simulink model "Filialist_PORTSDONE"  (R2019b)
settings: Solver=FixedStepAuto  StartTime=0.0  StopTime=inf  RelTol=1e-3
libraries: vexarmcortexlib x26, vexcommonlib x7
settings Model: ExtModeTrigDuration=25  Creator=nicoa  LastModifiedBy=nicoa
settings OptimizationCC: EnhancedBackFolding=on  PassReuseOutputArgsAs=Individual arguments  ZeroExternalMemoryAtStartup=off  ZeroInternalMemoryAtStartup=off  MaxStackSize=64  OptimizeBlockOrder=speed  DifferentSizesBufferReuse=on  OptimizationCustomize=off  EfficientTunableParamExpr=on
settings DebuggingCC: ParameterTunabilityLossMsg=error
settings HardwareCC: ProdBitPerPointer=32  ProdBitPerSizeT=32  ProdBitPerPtrDiffT=32  ProdLargestAtomicInteger=Long  ProdLargestAtomicFloat=Double  ProdWordSize=32  ProdHWDeviceType=ARM Compatible->ARM Cortex
settings SFSimCC: MATLABDynamicMemAlloc=off
settings RTWCC: SystemTargetFile=ert.tlc  HardwareBoard=ARM Cortex-based VEX Microcontroller  TLCOptions="-aInlineSetEventsForThisBaseRateFcn=TLC_FALSE -aSuppressMultiTaskScheduler=TLC_FALSE  -aRateBasedStepFcn=0"  TemplateMakefile=ert_default_tmf  GenerateReport=on  Toolchain=GNU Tools for VEX ARM Cortex  IncludeHyperlinkInReport=on  LaunchReport=on  GenerateTraceInfo=on  GenerateTraceReport=on  GenerateTraceReportSl=on  GenerateTraceReportSf=on  GenerateTraceReportEml=on
settings CodeAppCC: ForceParamTrailComments=on  IgnoreCustomStorageClasses=off  OperatorAnnotations=on  SimulinkDataObjDesc=on  SFDataObjDesc=on  InsertBlockDesc=on

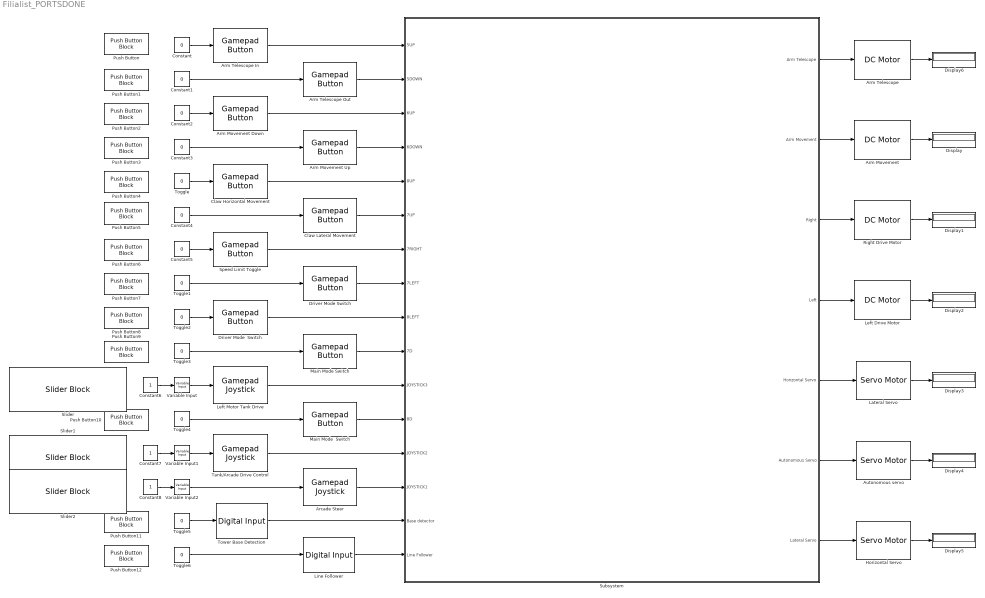
== system Filialist_PORTSDONE ==
  "Arcade Steer " : vexarmcortexlib/Gamepad/Gamepad Joystick  joystick=1  chan=1  SimulationIn=on  SampleTime=0.02
      settings: SourceProductName=Simulink Coder Support Package for ARM Cortex-based VEX Microcontroller  SourceProductBaseCode=EC_VEX_MICRO
  Arm Movement : vexarmcortexlib/Actuators/DC Motor  motor=6  scaleFactor=1/13.5  SimulationOut=on
      settings: SourceProductName=Simulink Coder Support Package for ARM Cortex-based VEX Microcontroller  SourceProductBaseCode=EC_VEX_MICRO
  Arm Movement Down : vexarmcortexlib/Gamepad/Gamepad Button  joystick=1  chan=6  button56=Down  button78=Down  SimulationIn=on  SampleTime=0.02
      settings: SourceProductName=Simulink Coder Support Package for ARM Cortex-based VEX Microcontroller  SourceProductBaseCode=EC_VEX_MICRO
  Arm Movement Up : vexarmcortexlib/Gamepad/Gamepad Button  joystick=1  chan=6  button56=Up  button78=Down  SimulationIn=on  SampleTime=0.02
      settings: SourceProductName=Simulink Coder Support Package for ARM Cortex-based VEX Microcontroller  SourceProductBaseCode=EC_VEX_MICRO
  Arm Telescope : vexarmcortexlib/Actuators/DC Motor  motor=2  scaleFactor=1/13.5  SimulationOut=on
      settings: SourceProductName=Simulink Coder Support Package for ARM Cortex-based VEX Microcontroller  SourceProductBaseCode=EC_VEX_MICRO
  Arm Telescope In : vexarmcortexlib/Gamepad/Gamepad Button  joystick=1  chan=5  button56=Down  button78=Down  SimulationIn=on  SampleTime=0.02
      settings: SourceProductName=Simulink Coder Support Package for ARM Cortex-based VEX Microcontroller  SourceProductBaseCode=EC_VEX_MICRO
  Arm Telescope Out : vexarmcortexlib/Gamepad/Gamepad Button  joystick=1  chan=5  button56=Up  button78=Down  SimulationIn=on  SampleTime=0.02
      settings: SourceProductName=Simulink Coder Support Package for ARM Cortex-based VEX Microcontroller  SourceProductBaseCode=EC_VEX_MICRO
  Autonomous servo : vexarmcortexlib/Actuators/Servo Motor  motor=5  scaleFactor=60/127  SimulationOut=on
      settings: SourceProductName=Simulink Coder Support Package for ARM Cortex-based VEX Microcontroller  SourceProductBaseCode=EC_VEX_MICRO
  Claw Horizontal Movement : vexarmcortexlib/Gamepad/Gamepad Button  joystick=1  chan=8  button56=Up  button78=Up  SimulationIn=on  SampleTime=0.02
      settings: SourceProductName=Simulink Coder Support Package for ARM Cortex-based VEX Microcontroller  SourceProductBaseCode=EC_VEX_MICRO
  Claw Lateral Movement : vexarmcortexlib/Gamepad/Gamepad Button  joystick=1  chan=7  button56=Up  button78=Up  SimulationIn=on  SampleTime=0.02
      settings: SourceProductName=Simulink Coder Support Package for ARM Cortex-based VEX Microcontroller  SourceProductBaseCode=EC_VEX_MICRO
  Constant{,1..5} (6 alike) : Constant  Value=0
  Constant6 : Constant
  Constant7 : Constant
  Constant8 : Constant
  Display{,1..6} (7 alike) : Display
  Driver Mode  Switch : vexarmcortexlib/Gamepad/Gamepad Button  joystick=1  chan=8  button56=Up  button78=Left  SimulationIn=on  SampleTime=0.02
      settings: SourceProductName=Simulink Coder Support Package for ARM Cortex-based VEX Microcontroller  SourceProductBaseCode=EC_VEX_MICRO
  Driver Mode Switch : vexarmcortexlib/Gamepad/Gamepad Button  joystick=1  chan=7  button56=Up  button78=Left  SimulationIn=on  SampleTime=0.02
      settings: SourceProductName=Simulink Coder Support Package for ARM Cortex-based VEX Microcontroller  SourceProductBaseCode=EC_VEX_MICRO
  Horizontal Servo : vexarmcortexlib/Actuators/Servo Motor  motor=3  scaleFactor=60/127  SimulationOut=on
      settings: SourceProductName=Simulink Coder Support Package for ARM Cortex-based VEX Microcontroller  SourceProductBaseCode=EC_VEX_MICRO
  Lateral Servo : vexarmcortexlib/Actuators/Servo Motor  motor=8  scaleFactor=60/127  SimulationOut=on
      settings: SourceProductName=Simulink Coder Support Package for ARM Cortex-based VEX Microcontroller  SourceProductBaseCode=EC_VEX_MICRO
  "Left Drive Motor " : vexarmcortexlib/Actuators/DC Motor  motor=9  scaleFactor=1/13.5  SimulationOut=on
      settings: SourceProductName=Simulink Coder Support Package for ARM Cortex-based VEX Microcontroller  SourceProductBaseCode=EC_VEX_MICRO
  Left Motor Tank Drive : vexarmcortexlib/Gamepad/Gamepad Joystick  joystick=1  chan=3  SimulationIn=on  SampleTime=0.02
      settings: SourceProductName=Simulink Coder Support Package for ARM Cortex-based VEX Microcontroller  SourceProductBaseCode=EC_VEX_MICRO
  Line Follower : vexarmcortexlib/Sensors/Digital Input  inChan=1  SimulationIn=on  SampleTime=0.2
      settings: SourceProductName=Simulink Coder Support Package for ARM Cortex-based VEX Microcontroller  SourceProductBaseCode=EC_VEX_MICRO
  Main Mode  Switch : vexarmcortexlib/Gamepad/Gamepad Button  joystick=1  chan=8  button56=Up  button78=Down  SimulationIn=on  SampleTime=0.02
      settings: SourceProductName=Simulink Coder Support Package for ARM Cortex-based VEX Microcontroller  SourceProductBaseCode=EC_VEX_MICRO
  Main Mode Switch : vexarmcortexlib/Gamepad/Gamepad Button  joystick=1  chan=7  button56=Up  button78=Down  SimulationIn=on  SampleTime=0.02
      settings: SourceProductName=Simulink Coder Support Package for ARM Cortex-based VEX Microcontroller  SourceProductBaseCode=EC_VEX_MICRO
  Push Button{,1..12} (13 alike) : PushButtonBlock
  Right Drive Motor : vexarmcortexlib/Actuators/DC Motor  motor=4  scaleFactor=1/13.5  SimulationOut=on
      settings: SourceProductName=Simulink Coder Support Package for ARM Cortex-based VEX Microcontroller  SourceProductBaseCode=EC_VEX_MICRO
  Slider : SliderBlock  LabelPosition=Hide  ScaleMin=-127  ScaleMax=127
  Slider1 : SliderBlock  LabelPosition=Hide  ScaleMin=-127  ScaleMax=127
  Slider2 : SliderBlock  LabelPosition=Hide  ScaleMin=-127  ScaleMax=127
  Speed Limit Toggle : vexarmcortexlib/Gamepad/Gamepad Button  joystick=1  chan=7  button56=Up  button78=Right  SimulationIn=on  SampleTime=0.02
      settings: SourceProductName=Simulink Coder Support Package for ARM Cortex-based VEX Microcontroller  SourceProductBaseCode=EC_VEX_MICRO
  Subsystem : Subsystem
  Tank/Arcade Drive Control : vexarmcortexlib/Gamepad/Gamepad Joystick  joystick=1  chan=2  SimulationIn=on  SampleTime=0.02
      settings: SourceProductName=Simulink Coder Support Package for ARM Cortex-based VEX Microcontroller  SourceProductBaseCode=EC_VEX_MICRO
  Toggle{,1..6} (7 alike) : Constant  Value=0
      settings: OpenFcn=|
      | if strcmp('0',get_param(gcb, 'Value'))                        set_param(gcb, 'Value', '1');
      | else
      |             set_param(gcb, 'Value', '0');
      | end
  Tower Base Detection : vexarmcortexlib/Sensors/Digital Input  inChan=11  SimulationIn=on  SampleTime=0.2
      settings: SourceProductName=Simulink Coder Support Package for ARM Cortex-based VEX Microcontroller  SourceProductBaseCode=EC_VEX_MICRO
  Variable Input : vexarmcortexlib/Utilities/Variable Input  low=-127  gain=0  high=127
      settings: SourceProductName=Simulink Coder Support Package for ARM Cortex-based VEX Microcontroller  SourceProductBaseCode=EC_VEX_MICRO
  Variable Input1 : vexarmcortexlib/Utilities/Variable Input  low=-127  gain=0  high=127
      settings: SourceProductName=Simulink Coder Support Package for ARM Cortex-based VEX Microcontroller  SourceProductBaseCode=EC_VEX_MICRO
  Variable Input2 : vexarmcortexlib/Utilities/Variable Input  low=-127  gain=0  high=127
      settings: SourceProductName=Simulink Coder Support Package for ARM Cortex-based VEX Microcontroller  SourceProductBaseCode=EC_VEX_MICRO
  wires:
  Main Mode  Switch/1 -> Subsystem/12(8D)
  Main Mode Switch/1 -> Subsystem/10(7D)
  Subsystem/4(Left) -> "Left Drive Motor "/1
  Subsystem/6(Autonomous Servo) -> Autonomous servo/1
  Tower Base Detection/1 -> Subsystem/15(Base detector)
  Line Follower/1 -> Subsystem/16(Line Follower)
  Driver Mode  Switch/1 -> Subsystem/9(8LEFT)
  Driver Mode Switch/1 -> Subsystem/8(7LEFT)
  Speed Limit Toggle/1 -> Subsystem/7(7RIGHT)
  Tank/Arcade Drive Control/1 -> Subsystem/13(JOYSTICK2)
  Left Motor Tank Drive/1 -> Subsystem/11(JOYSTICK3)
  "Arcade Steer "/1 -> Subsystem/14(JOYSTICK1)
  Subsystem/3(Right) -> Right Drive Motor/1
  Subsystem/7(Lateral Servo) -> Horizontal Servo/1
  Subsystem/5(Horizontal Servo) -> Lateral Servo/1
  Claw Lateral Movement/1 -> Subsystem/6(7UP)
  Claw Horizontal Movement/1 -> Subsystem/5(8UP)
  Subsystem/2(Arm Movement) -> Arm Movement/1
  Arm Movement Up/1 -> Subsystem/4(6DOWN)
  Arm Movement Down/1 -> Subsystem/3(6UP)
  Subsystem/1(Arm Telescope) -> Arm Telescope/1
  Arm Telescope Out/1 -> Subsystem/2(5DOWN)
  Arm Telescope In/1 -> Subsystem/1(5UP)
  Arm Movement/1 -> Display/1
  Right Drive Motor/1 -> Display1/1
  "Left Drive Motor "/1 -> Display2/1
  Lateral Servo/1 -> Display3/1
  Autonomous servo/1 -> Display4/1
  Horizontal Servo/1 -> Display5/1
  Arm Telescope/1 -> Display6/1
  Constant/1 -> Arm Telescope In/1
  Constant1/1 -> Arm Telescope Out/1
  Constant2/1 -> Arm Movement Down/1
  Constant3/1 -> Arm Movement Up/1
  Toggle/1 -> Claw Horizontal Movement/1
  Constant4/1 -> Claw Lateral Movement/1
  Constant5/1 -> Speed Limit Toggle/1
  Toggle1/1 -> Driver Mode Switch/1
  Toggle2/1 -> Driver Mode  Switch/1
  Toggle3/1 -> Main Mode Switch/1
  Constant6/1 -> Variable Input/1
  Variable Input/1 -> Left Motor Tank Drive/1
  Variable Input1/1 -> Tank/Arcade Drive Control/1
  Constant7/1 -> Variable Input1/1
  Variable Input2/1 -> "Arcade Steer "/1
  Constant8/1 -> Variable Input2/1
  Toggle4/1 -> Main Mode  Switch/1
  Toggle5/1 -> Tower Base Detection/1
  Toggle6/1 -> Line Follower/1

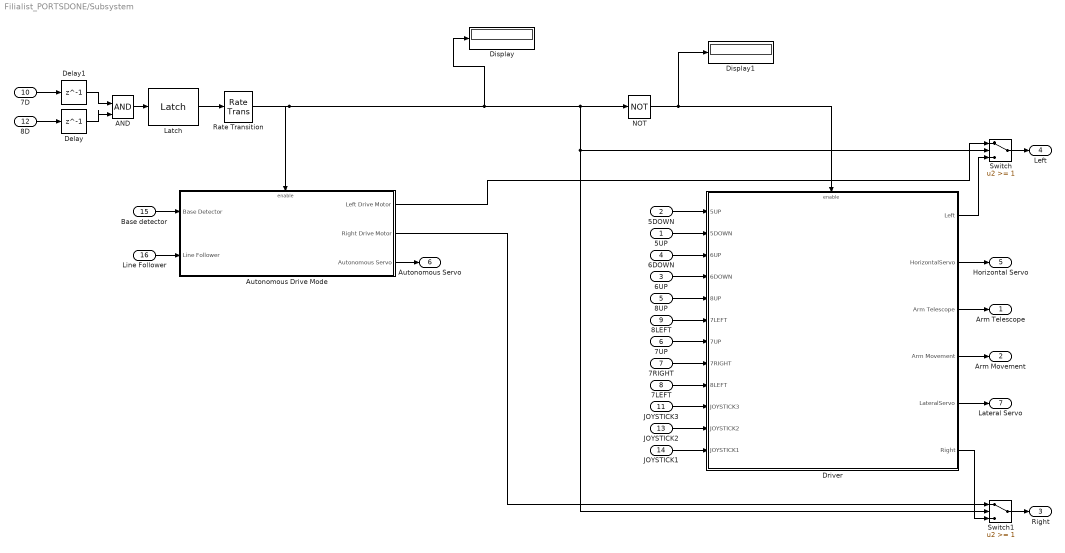
== system Filialist_PORTSDONE/Subsystem ==
  5UP : Inport
  5DOWN : Inport  Port=2
  6UP : Inport  Port=3
  6DOWN : Inport  Port=4
  8UP : Inport  Port=5
  7UP : Inport  Port=6
  7RIGHT : Inport  Port=7
  7LEFT : Inport  Port=8
  8LEFT : Inport  Port=9
  7D : Inport  Port=10
  JOYSTICK3 : Inport  Port=11
  8D : Inport  Port=12
  JOYSTICK2 : Inport  Port=13
  JOYSTICK1 : Inport  Port=14
  Base detector : Inport  Port=15
  Line Follower : Inport  Port=16
  "AND " : Logic  IconShape=distinctive  AllPortsSameDT=off  OutDataTypeStr=boolean
  Autonomous Drive Mode : Subsystem
  Delay : Delay  DelayLength=1  InitialCondition=0  SampleTime=1
  Delay1 : Delay  DelayLength=1  InitialCondition=0  SampleTime=1
  Display : Display
  Display1 : Display
  Driver : Subsystem  TreatAsAtomicUnit=on
  Latch : vexcommonlib/Latch  output0=off  BlockPlatform=vexarmcortex
      settings: SourceProductName=Simulink Coder Support Package for ARM Cortex-based VEX Microcontroller  SourceProductBaseCode=EC_VEX_MICRO
  NOT : Logic  Operator=NOT  IconShape=distinctive  AllPortsSameDT=off  OutDataTypeStr=boolean
  Rate Transition : RateTransition
  Switch : Switch  Threshold=1
  Switch1 : Switch  Threshold=1
  Arm Telescope : Outport
  Arm Movement : Outport  Port=2
  Right : Outport  Port=3
  Left : Outport  Port=4
  Horizontal Servo : Outport  Port=5
  Autonomous Servo : Outport  Port=6
  Lateral Servo : Outport  Port=7
  wires:
  "AND "/1 -> Latch/1
  Delay1/1 -> "AND "/1
  Latch/1 -> Rate Transition/1
  7D/1 -> Delay1/1
  Delay/1 -> "AND "/2
  8D/1 -> Delay/1
  Autonomous Drive Mode/3(Autonomous Servo) -> Autonomous Servo/1
  Rate Transition/1 -> Autonomous Drive Mode/Enable, NOT/1, Switch1/2, Switch/2, Display/1
  NOT/1 -> Driver/Enable, Display1/1
  Autonomous Drive Mode/1(Left Drive Motor) -> Switch/1
  Switch/1 -> Left/1
  Autonomous Drive Mode/2(Right Drive Motor) -> Switch1/1
  Switch1/1 -> Right/1
  Line Follower/1 -> Autonomous Drive Mode/2(Line Follower)
  Base detector/1 -> Autonomous Drive Mode/1(Base Detector)
  7LEFT/1 -> Driver/9(8LEFT)
  8LEFT/1 -> Driver/6(7LEFT)
  7RIGHT/1 -> Driver/8(7RIGHT)
  JOYSTICK3/1 -> Driver/10(JOYSTICK3)
  JOYSTICK2/1 -> Driver/11(JOYSTICK2)
  JOYSTICK1/1 -> Driver/12(JOYSTICK1)
  Driver/5(LateralServo) -> Lateral Servo/1
  Driver/2(HorizontalServo) -> Horizontal Servo/1
  8UP/1 -> Driver/5(8UP)
  7UP/1 -> Driver/7(7UP)
  Driver/4(Arm Movement) -> Arm Movement/1
  6UP/1 -> Driver/4(6DOWN)
  6DOWN/1 -> Driver/3(6UP)
  Driver/3(Arm Telescope) -> Arm Telescope/1
  5UP/1 -> Driver/2(5DOWN)
  5DOWN/1 -> Driver/1(5UP)
  Driver/6(Right) -> Switch1/3
  Driver/1(Left) -> Switch/3

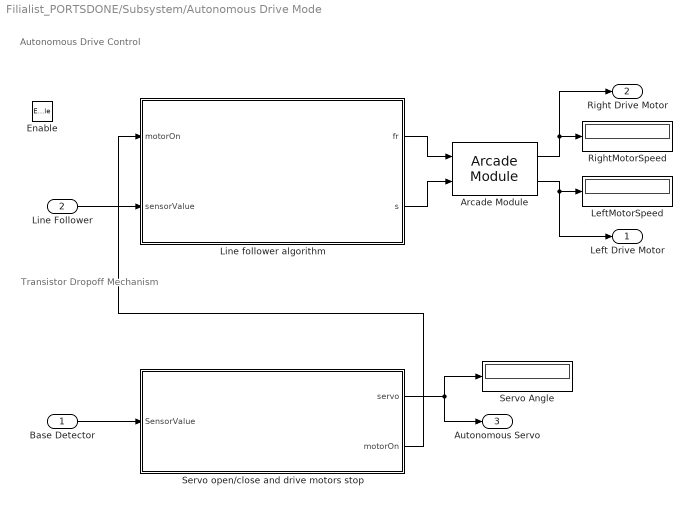
== system Filialist_PORTSDONE/Subsystem/Autonomous Drive Mode ==
  note: Transistor Dropoff Mechanism
  note: Autonomous Drive Control
  Base Detector : Inport
  Line Follower : Inport  Port=2
  Enable : EnablePort
  Arcade Module : vexcommonlib/Arcade Module  BlockPlatform=vexarmcortex
      settings: SourceProductName=Simulink Coder Support Package for ARM Cortex-based VEX Microcontroller  SourceProductBaseCode=EC_VEX_MICRO
  LeftMotorSpeed : Display
  Line follower algorithm : Stateflow chart  TreatAsAtomicUnit=on
  RightMotorSpeed : Display
  Servo Angle : Display
  Servo open/close and drive motors stop : Stateflow chart  TreatAsAtomicUnit=on
  Left Drive Motor : Outport
  Right Drive Motor : Outport  Port=2
  Autonomous Servo : Outport  Port=3
  wires:
  Base Detector/1 -> Servo open/close and drive motors stop/1(SensorValue)
  Line Follower/1 -> Line follower algorithm/2(sensorValue)
  Line follower algorithm/2(s) -> Arcade Module/2
  Line follower algorithm/1(fr) -> Arcade Module/1
  Arcade Module/1 -> RightMotorSpeed/1, Right Drive Motor/1
  Arcade Module/2 -> LeftMotorSpeed/1, Left Drive Motor/1
  Servo open/close and drive motors stop/1(servo) -> Autonomous Servo/1, Servo Angle/1
  Servo open/close and drive motors stop/2(motorOn) -> Line follower algorithm/1(motorOn)

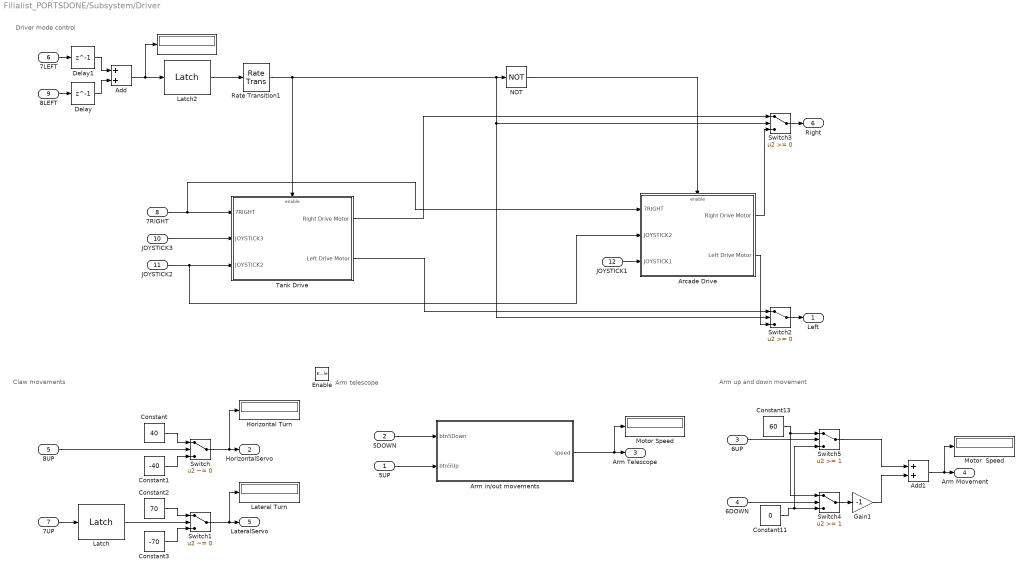
== system Filialist_PORTSDONE/Subsystem/Driver ==
  note: Arm telescope
  note: Claw movements
  note: Arm up and down movement
  note: Driver mode control
  5UP : Inport
  5DOWN : Inport  Port=2
  6UP : Inport  Port=3
  6DOWN : Inport  Port=4
  8UP : Inport  Port=5
  7LEFT : Inport  Port=6
  7UP : Inport  Port=7
  7RIGHT : Inport  Port=8
  8LEFT : Inport  Port=9
  JOYSTICK3 : Inport  Port=10
  JOYSTICK2 : Inport  Port=11
  JOYSTICK1 : Inport  Port=12
  Enable : EnablePort
  " " : Display
  Add : Sum
  Add1 : Sum
  "Arcade Drive " : Subsystem  TreatAsAtomicUnit=on
  Arm in/out movements : Stateflow chart  BlockKeywords=__PRM__SERIALIZED__DATA__:Stateflow Chart,Stateflow Diagram  TreatAsAtomicUnit=on
  Constant : Constant  Value=40
  Constant1 : Constant  Value=-40
  Constant11 : Constant  Value=0
  Constant13 : Constant  Value=60
  Constant2 : Constant  Value=70
  Constant3 : Constant  Value=-70
  Delay : Delay  DelayLength=1  InitialCondition=0  SampleTime=1
  Delay1 : Delay  DelayLength=1  InitialCondition=0  SampleTime=1
  Gain1 : Gain  Gain=-1
  Horizontal Turn : Display
  Latch : vexcommonlib/Latch  output0=off  BlockPlatform=vexarmcortex
      settings: SourceProductName=Simulink Coder Support Package for ARM Cortex-based VEX Microcontroller  SourceProductBaseCode=EC_VEX_MICRO
  Latch2 : vexcommonlib/Latch  output0=off  BlockPlatform=vexarmcortex
      settings: SourceProductName=Simulink Coder Support Package for ARM Cortex-based VEX Microcontroller  SourceProductBaseCode=EC_VEX_MICRO
  Lateral Turn : Display
  Motor  Speed : Display
  Motor Speed : Display
  NOT : Logic  Operator=NOT  IconShape=distinctive  AllPortsSameDT=off  OutDataTypeStr=boolean
  Rate Transition1 : RateTransition
  Switch : Switch  Criteria=u2 ~= 0
  Switch1 : Switch  Criteria=u2 ~= 0
  Switch2 : Switch
  Switch3 : Switch
  Switch4 : Switch  Threshold=1
  Switch5 : Switch  Threshold=1
  "Tank Drive " : Subsystem  TreatAsAtomicUnit=on
  Left : Outport
  HorizontalServo : Outport  Port=2
  Arm Telescope : Outport  Port=3
  Arm Movement : Outport  Port=4
  LateralServo : Outport  Port=5
  Right : Outport  Port=6
  wires:
  Rate Transition1/1 -> Switch2/2, Switch3/2, NOT/1, "Tank Drive "/Enable
  7LEFT/1 -> Delay1/1
  NOT/1 -> "Arcade Drive "/Enable
  Delay1/1 -> Add/1
  Delay/1 -> Add/2
  Latch2/1 -> Rate Transition1/1
  Add/1 -> " "/1, Latch2/1
  8LEFT/1 -> Delay/1
  JOYSTICK3/1 -> "Tank Drive "/2(JOYSTICK3)
  JOYSTICK2/1 -> "Tank Drive "/3(JOYSTICK2), "Arcade Drive "/2(JOYSTICK2)
  JOYSTICK1/1 -> "Arcade Drive "/3(JOYSTICK1)
  Constant/1 -> Switch/1
  7UP/1 -> Latch/1
  Latch/1 -> Switch1/2
  Switch/1 -> Horizontal Turn/1, HorizontalServo/1
  Constant1/1 -> Switch/3
  Switch1/1 -> Lateral Turn/1, LateralServo/1
  Constant2/1 -> Switch1/1
  Constant3/1 -> Switch1/3
  Switch4/1 -> Gain1/1
  Constant11/1 -> Switch5/3, Switch4/3
  6DOWN/1 -> Switch4/2
  6UP/1 -> Switch5/2
  Constant13/1 -> Switch5/1, Switch4/1
  Add1/1 -> Motor  Speed/1, Arm Movement/1
  5UP/1 -> Arm in/out movements/2(btn5Up)
  Arm in/out movements/1(speed) -> Motor Speed/1, Arm Telescope/1
  5DOWN/1 -> Arm in/out movements/1(btn5Down)
  Switch2/1 -> Left/1
  "Arcade Drive "/2(Left Drive Motor) -> Switch2/3
  Switch3/1 -> Right/1
  "Arcade Drive "/1(Right Drive Motor) -> Switch3/3
  7RIGHT/1 -> "Tank Drive "/1(7RIGHT), "Arcade Drive "/1(7RIGHT)
  "Tank Drive "/2(Left Drive Motor) -> Switch2/1
  "Tank Drive "/1(Right Drive Motor) -> Switch3/1
  Switch5/1 -> Add1/1
  Gain1/1 -> Add1/2
  8UP/1 -> Switch/2

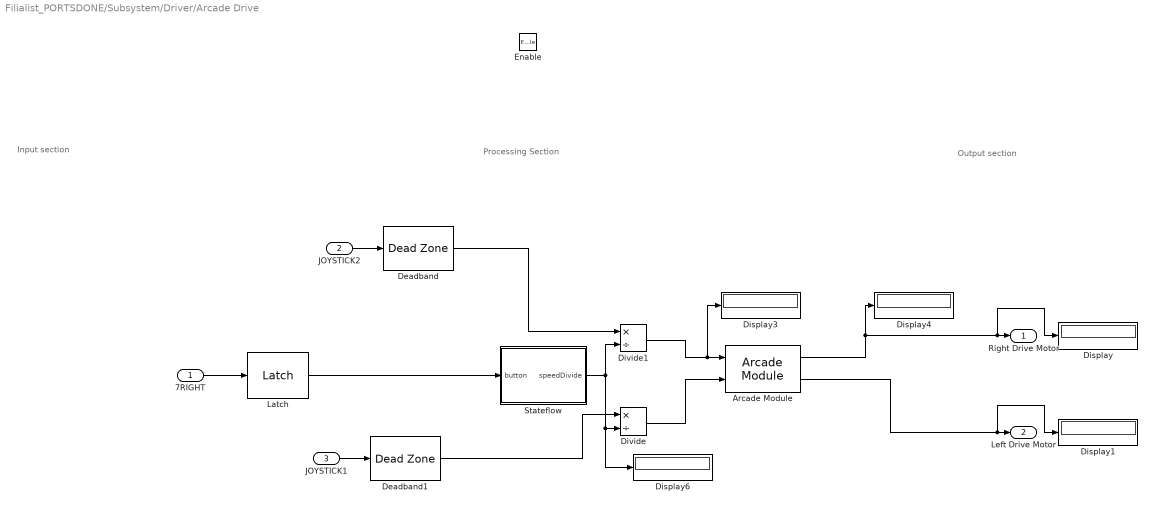
== system Filialist_PORTSDONE/Subsystem/Driver/Arcade Drive  ==
  note: Output section
  note: Processing Section
  note: Input section
  7RIGHT : Inport
  JOYSTICK2 : Inport  Port=2
  JOYSTICK1 : Inport  Port=3
  Enable : EnablePort
  Arcade Module : vexcommonlib/Arcade Module  BlockPlatform=vexarmcortex
      settings: SourceProductName=Simulink Coder Support Package for ARM Cortex-based VEX Microcontroller  SourceProductBaseCode=EC_VEX_MICRO
  Deadband : DeadZone  LowerValue=-5  UpperValue=5  SaturateOnIntegerOverflow=on
  Deadband1 : DeadZone  LowerValue=-5  UpperValue=5  SaturateOnIntegerOverflow=on
  Display{,1,3..4,6} (5 alike) : Display
  Divide : Product  Inputs=*/
  Divide1 : Product  Inputs=*/
  Latch : vexcommonlib/Latch  output0=off  BlockPlatform=vexarmcortex
      settings: SourceProductName=Simulink Coder Support Package for ARM Cortex-based VEX Microcontroller  SourceProductBaseCode=EC_VEX_MICRO
  Stateflow : Stateflow chart  TreatAsAtomicUnit=on
  Right Drive Motor : Outport
  Left Drive Motor : Outport  Port=2
  wires:
  JOYSTICK1/1 -> Deadband1/1
  JOYSTICK2/1 -> Deadband/1
  7RIGHT/1 -> Latch/1
  Stateflow/1(speedDivide) -> Display6/1, Divide/2, Divide1/2
  Deadband/1 -> Divide1/1
  Deadband1/1 -> Divide/1
  Divide/1 -> Arcade Module/2
  Divide1/1 -> Display3/1, Arcade Module/1
  Arcade Module/1 -> Display/1, Right Drive Motor/1, Display4/1
  Arcade Module/2 -> Display1/1, Left Drive Motor/1
  Latch/1 -> Stateflow/1(button)

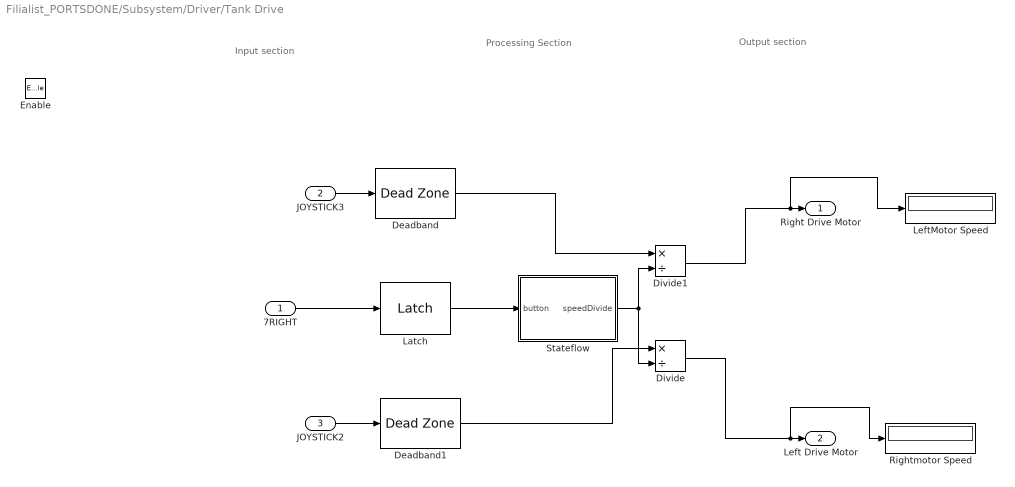
== system Filialist_PORTSDONE/Subsystem/Driver/Tank Drive  ==
  note: Output section
  note: Processing Section
  note: Input section
  7RIGHT : Inport
  JOYSTICK3 : Inport  Port=2
  JOYSTICK2 : Inport  Port=3
  Enable : EnablePort
  Deadband : DeadZone  LowerValue=-5  UpperValue=5  SaturateOnIntegerOverflow=on
  Deadband1 : DeadZone  LowerValue=-5  UpperValue=5  SaturateOnIntegerOverflow=on
  Divide : Product  Inputs=*/
  Divide1 : Product  Inputs=*/
  Latch : vexcommonlib/Latch  output0=off  BlockPlatform=vexarmcortex
      settings: SourceProductName=Simulink Coder Support Package for ARM Cortex-based VEX Microcontroller  SourceProductBaseCode=EC_VEX_MICRO
  LeftMotor Speed : Display
  Rightmotor Speed : Display
  Stateflow : Stateflow chart  TreatAsAtomicUnit=on
  Right Drive Motor : Outport
  Left Drive Motor : Outport  Port=2
  wires:
  JOYSTICK3/1 -> Deadband/1
  7RIGHT/1 -> Latch/1
  Latch/1 -> Stateflow/1(button)
  Stateflow/1(speedDivide) -> Divide1/2, Divide/2
  Deadband/1 -> Divide1/1
  Deadband1/1 -> Divide/1
  Divide1/1 -> LeftMotor Speed/1, Right Drive Motor/1
  Divide/1 -> Rightmotor Speed/1, Left Drive Motor/1
  JOYSTICK2/1 -> Deadband1/1

== stateflow chart Filialist_PORTSDONE/Subsystem/Autonomous Drive Mode/Line follower algorithm ==
  state GO_RIGHT
    entry:
    fr = 50;
    s = -50;
  state GO_LEFT
    entry:
    fr = 50;
    s = 50;
  state STOPPED
    entry:
    fr = 0;
    s = 0;
  (default) -> GO_LEFT
  GO_LEFT -> GO_RIGHT [order 2] : [sensorValue == 1]
  GO_RIGHT -> GO_LEFT [order 2] : [sensorValue == 0]
  GO_LEFT -> STOPPED [order 1] : [motorOn == 0]
  GO_RIGHT -> STOPPED [order 1] : [motorOn == 0]
  data: fr output; s output; motorOn input; sensorValue input

== stateflow chart Filialist_PORTSDONE/Subsystem/Driver/Arcade Drive /Stateflow ==
  state Full_Speed
    entry:
    speedDivide = 1
  state Slow_Speed
    entry:
    speedDivide = 4
  (default) -> Full_Speed
  Full_Speed -> Slow_Speed : [button == 1]
  Slow_Speed -> Full_Speed : [button == 0]
  data: speedDivide output; button input

== stateflow chart Filialist_PORTSDONE/Subsystem/Driver/Tank Drive /Stateflow ==
  state Full_Speed
    entry:
    speedDivide = 1
  state Slow_Speed
    entry:
    speedDivide = 4
  (default) -> Full_Speed
  Full_Speed -> Slow_Speed : [button]
  Slow_Speed -> Full_Speed : [button == 0]
  data: speedDivide output; button input

== stateflow chart Filialist_PORTSDONE/Subsystem/Autonomous Drive Mode/Servo open//close and drive motors stop ==
  state move
    entry:
    servo = 0;
    motorOn = 1;
  state Stop
    entry:
    servo = 67;
    motorOn = 0;
  state off
    entry:
    servo = 0;
    motorOn = 0;
  (default) -> move
  move -> Stop : [SensorValue == 1]
  Stop -> off : [after(4,sec)]
  data: SensorValue input; servo output; motorOn output

== stateflow chart Filialist_PORTSDONE/Subsystem/Driver/Arm in//out movements ==
  state ARMDOWN
    entry:
    speed = -40;
  state STOPPED
    entry:
    speed = 0;
  state ARMUP
    entry:
    speed = 40;
  (default) -> STOPPED
  STOPPED -> ARMUP [order 1] : [btn5Down == 0 && btn5Up == 1 ]
  STOPPED -> ARMDOWN [order 2] : [btn5Down == 1 && btn5Up == 0]
  ARMDOWN -> STOPPED [order 2] : [btn5Down == 0]
  ARMUP -> STOPPED [order 2] : [btn5Up == 0]
  ARMDOWN -> STOPPED [order 1] : [btn5Down == 1 && btn5Up == 1]
  ARMUP -> STOPPED [order 1] : [btn5Down == 1 && btn5Up == 1]
  data: btn5Down input; btn5Up input; speed output
